simulink model "SingleSine"  (R2022b)
settings: Solver=VariableStepAuto  StartTime=0.0  StopTime=10.0  RelTol=1e-3
StartFcn:
  | lib_name = '';
  | 
  | if strcmp(computer, 'PCWIN')
  |   lib_name = 'dxl_x86_c';
  | elseif strcmp(computer, 'PCWIN64')
  |   lib_name = 'dxl_x64_c';
  | elseif strcmp(computer, 'GLNX86')
  |   lib_name = 'libdxl_x86_c';
  | elseif strcmp(computer, 'GLNXA64')
  |   lib_name = 'libdxl_x64_c';
  | elseif strcmp(computer, 'MACI64')
  |   lib_name = 'libdxl_mac_c';
  | end
  | 
  | % Load Libraries
  | if ~libisloaded(lib_name)
  |     [notfound, warnings] = loadlibrary(lib_name, 'dynamixel_sdk.h', 'addheader', 'port_handler.h', 'addheader', 'packet_handler.h');
  | end
  | My_DXL = 'X_SERIES'; % X330, X430, X540, 2X430
  | 
  | % Control table address and data to Read/Write for my DYNAMIXEL, My_DXL, in use.
  |         ADDR_TORQUE_ENABLE          = 64;
  |         ADDR_GOAL_CURRENT           = 102;
  |         ADDR_GOAL_POSITION          = 116;
  |         ADDR_PRESENT_POSITION       = 132;
  |         ADDR_PRESENT_CURRENT        = 126;
  |         ADDR_CURRENT_LIMIT          = 38;
  |         DXL_MINIMUM_POSITION_VALUE  = 1000; % Dynamixel will rotate between this value
  |         DXL_MAXIMUM_POSITION_VALUE  = 3000; % and this value (note that the Dynamixel would not move when the position value is out of movable range. Check e-manual about the range of the Dynamixel you use.)
  |         BAUDRATE                    = 1000000;
  | 
  | % DYNAMIXEL Protocol Version (1.0 / 2.0)
  | % https://emanual.robotis.com/docs/en/dxl/protocol2/
  | PROTOCOL_VERSION            = 2.0;
  | 
  | % Factory default ID of all DYNAMIXEL is 1
  | DXL_ID                      = 11;
  | 
  | % Use the actual port assigned to the U2D2.
  | % ex) Windows: 'COM*', Linux: '/dev/ttyUSB*', Mac: '/dev/tty.usbserial-*'
  | DEVICENAME                  = 'COM6';
  | 
  | % Common Control Table Address and Data
  | ADDR_OPERATING_MODE         = 11;
  | OPERATING_MODE              = 0;            % value for operating mode for position control
  | TORQUE_ENABLE               = 1;            % Value for enabling the torque
  | TORQUE_DISABLE              = 0;            % Value for disabling the torque
  | DXL_MOVING_STATUS_THRESHOLD = 20;           % Dynamixel moving status threshold
  | 
  | COMM_SUCCESS                = 0;            % Communication Success result value
  | COMM_TX_FAIL                = -1001;        % Communication Tx Failed
  | 
  | % Initialize PortHandler Structs
  | % Set the port path
  | % Get methods and members of PortHandlerLinux or PortHandlerWindows
  | port_num = portHandler(DEVICENAME);
  | 
  | % Initialize PacketHandler Structs
  | packetHandler();
  | 
  | index = 1;
  | dxl_comm_result = COMM_TX_FAIL;           % Communication result
  | dxl_goal_position = [1000 1500 2000];         % Goal position    DXL_MINIMUM_POSITION_VALUE  DXL_MAXIMUM_POSITION_VALUE
  | 
  | dxl_error = 0;                              % Dynamixel error
  | dxl_present_position = 0;                   % Present position
  | 
  | 
  | % Open port
  | if (openPort(port_num))
  |     fprintf('Succeeded to open the port!\n');
  | else
  |     unloadlibrary(lib_name);
  |     fprintf('Failed to open the port!\n');
  |     input('Press any key to terminate...\n');
  |     return;
  | end
  | 
  | 
  | % Set port baudrate
  | if (setBaudRate(port_num, BAUDRATE))
  |     fprintf('Succeeded to change the baudrate!\n');
  | else
  |     unloadlibrary(lib_name);
  |     fprintf('Failed to change the baudrate!\n');
  |     input('Press any key to terminate...\n');
  |     return;
  | end
  | 
  | 
  | % Enable Dynamixel Torque
  | write1ByteTxRx(port_num, PROTOCOL_VERSION, DXL_ID, ADDR_TORQUE_ENABLE, TORQUE_ENABLE);
  | dxl_comm_result = getLastTxRxResult(port_num, PROTOCOL_VERSION);
  | dxl_error = getLastRxPacketError(port_num, PROTOCOL_VERSION);
  | if dxl_comm_result ~= COMM_SUCCESS
  |     fprintf('%s\n', getTxRxResult(PROTOCOL_VERSION, dxl_comm_result));
  | elseif dxl_error ~= 0
  |     fprintf('%s\n', getRxPacketError(PROTOCOL_VERSION, dxl_error));
  | else
  |     fprintf('Dynamixel has been successfully connected \n');
  | end
CloseFcn:
  | % Disable Dynamixel Torque
  | write1ByteTxRx(port_num, PROTOCOL_VERSION, DXL_ID, ADDR_TORQUE_ENABLE, TORQUE_DISABLE);
  | dxl_comm_result = getLastTxRxResult(port_num, PROTOCOL_VERSION);
  | dxl_error = getLastRxPacketError(port_num, PROTOCOL_VERSION);
  | if dxl_comm_result ~= COMM_SUCCESS
  |     fprintf('%s\n', getTxRxResult(PROTOCOL_VERSION, dxl_comm_result));
  | elseif dxl_error ~= 0
  |     fprintf('%s\n', getRxPacketError(PROTOCOL_VERSION, dxl_error));
  | end
  | 
  | % Close port
  | closePort(port_num);
  | 
  | % Unload Library
  | unloadlibrary(lib_name);
  | 
  | close all;
  | clear;
settings Model: Creator=Boog  LastModifiedBy=Boog

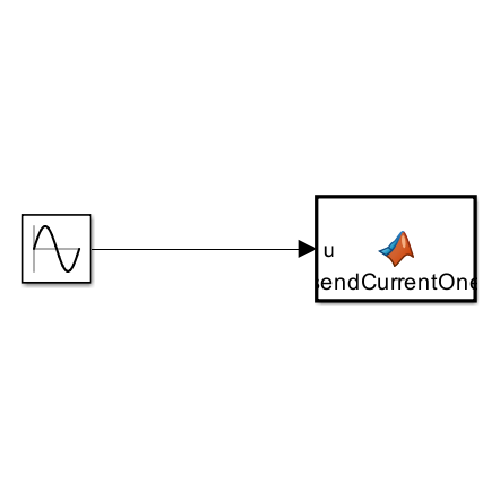
[thumbnail: Simulink's stored preview of the top-level diagram]
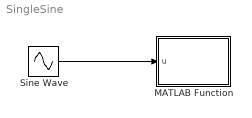
== system SingleSine ==
  MATLAB Function : MATLAB Function  TreatAsAtomicUnit=on
  Sine Wave : Sin  SampleTime=0
  wires:
  Sine Wave/1 -> MATLAB Function/1(u)

== matlab function SingleSine/MATLAB Function ==
  data: u input
function sendCurrentOne(u)
    PROTOCOL_VERSION    = 2.0;
    DXL_ID              = 11;
    ADDR_GOAL_CURRENT   = 102;
    COMM_SUCCESS                = 0;
    COMM_TX_FAIL                = -1001; 
    dxl_comm_result = COMM_TX_FAIL;
    port_num = 0;

    % 1.5A / 1.6 N-m
    
    % 0.9375 A/N-m
    
    % Current in Amps = 0.9375 * t[N-m]

    % Current in mA = Current in Amps * 1000

    % Current in Data = Current in mA / 2.69

    current_A = 0.9375 .* u;
    
    current_data = current_A .* 1000 ./ 2.69;
    
    % Write goal current
    write2ByteTxRx(port_num, PROTOCOL_VERSION, DXL_ID, ADDR_GOAL_CURRENT, typecast(int16(current_data(1)), 'uint16'));
    dxl_comm_result = getLastTxRxResult(port_num, PROTOCOL_VERSION);
    dxl_error = getLastRxPacketError(port_num, PROTOCOL_VERSION);
    if dxl_comm_result ~= COMM_SUCCESS
        fprintf('%s\n', getTxRxResult(PROTOCOL_VERSION, dxl_comm_result));
    elseif dxl_error ~= 0
        fprintf('%s\n', getRxPacketError(PROTOCOL_VERSION, dxl_error));
    end  
end
